simulink model "HumanActionModel"  (R2022b)
settings: Solver=VariableStepAuto  StartTime=0.0  StopTime=5  FixedStep=0.01  RelTol=1e-3
values from neighbouring files (symbols this model uses):
  uD = -0.1    [kavya.mat]
settings Model: Creator=abane  LastModifiedBy=chand

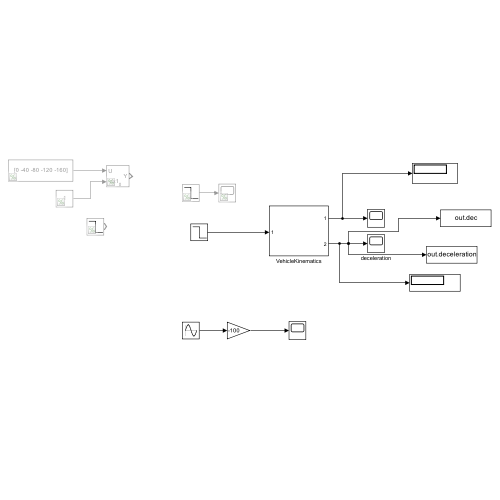
[thumbnail: Simulink's stored preview of the top-level diagram]
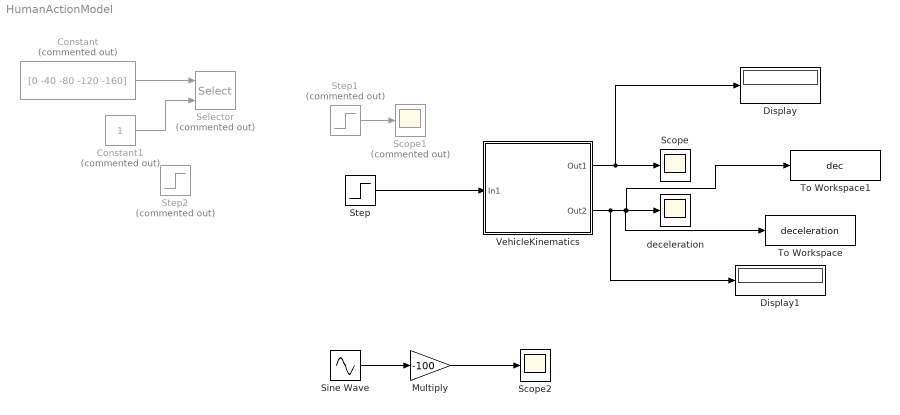
== system HumanActionModel ==
  Constant : Constant  Commented=on  Value=[0 -40 -80 -120 -160]
  Constant1 : Constant  Commented=on
  Display : Display
  Display1 : Display
  Multiply : Gain  Gain=-100
  Scope : Scope
  Scope1 : Scope  Commented=on
  Scope2 : Scope
  Selector : Selector  Commented=on  IndexMode=Zero-based  InputPortWidth=5  IndexOptions=Index vector (port)  Indices=[1 3]  OutputSizes=1
  Sine Wave : Sin  Amplitude=0.5  SampleTime=0
  Step : Step  Time=0.40692  After=-165  SampleTime=0
  Step1 : Step  Commented=on  Time=0.03461  After=-165  SampleTime=0
  Step2 : Step  Commented=on  Time=0.03461  After=-165  SampleTime=0
  To Workspace : ToWorkspace  VariableName=deceleration  SaveFormat=Structure With Time  SampleTime=-1
  To Workspace1 : ToWorkspace  VariableName=dec  SaveFormat=Structure With Time  SampleTime=-1
  VehicleKinematics : Subsystem
  deceleration : Scope
  wires:
  VehicleKinematics/1(Out1) -> Display/1, Scope/1
  VehicleKinematics/2(Out2) -> To Workspace/1, To Workspace1/1, deceleration/1, Display1/1
  Constant/1 -> Selector/1
  Constant1/1 -> Selector/2
  Sine Wave/1 -> Multiply/1
  Multiply/1 -> Scope2/1
  Step/1 -> VehicleKinematics/1(In1)
  Step1/1 -> Scope1/1

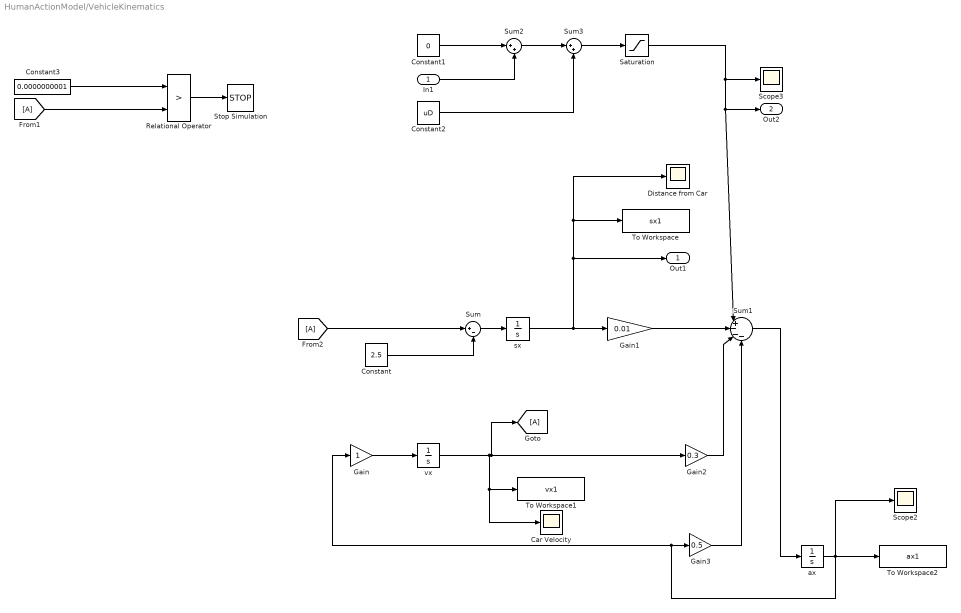
== system HumanActionModel/VehicleKinematics ==
  In1 : Inport
  Car Velocity : Scope
  Constant : Constant  Value=2.5
  Constant1 : Constant  Value=0
  Constant2 : Constant  Value=uD
  Constant3 : Constant  Value=0.0000000001
  Distance from Car : Scope
  From1 : From
  From2 : From
  Gain : Gain
  Gain1 : Gain  Gain=0.01
  Gain2 : Gain  Gain=0.3
  Gain3 : Gain  Gain=0.5
  Goto : Goto
  Relational Operator : RelationalOperator  Operator=>  OutDataTypeStr=boolean  RndMeth=Simplest  InputSameDT=off
  Saturation : Saturate  UpperLimit=0  LowerLimit=-165
  Scope2 : Scope
  Scope3 : Scope
  Stop Simulation : Stop
  Sum : Sum  Inputs=|+-
  Sum1 : Sum  Inputs=|+---
  Sum2 : Sum  Inputs=|++
  Sum3 : Sum  Inputs=|++
  To Workspace : ToWorkspace  VariableName=sx1  SaveFormat=Timeseries  SampleTime=-1
  To Workspace1 : ToWorkspace  VariableName=vx1  SaveFormat=Timeseries  SampleTime=-1
  To Workspace2 : ToWorkspace  VariableName=ax1  SaveFormat=Timeseries  SampleTime=-1
  ax : Integrator
  sx : Integrator  InitialCondition=-43.8
  vx : Integrator  InitialCondition=60
  Out1 : Outport
  Out2 : Outport  Port=2
  wires:
  Constant3/1 -> Relational Operator/1
  Relational Operator/1 -> Stop Simulation/1
  Sum/1 -> sx/1
  Gain/1 -> vx/1
  Constant1/1 -> Sum2/1
  Gain2/1 -> Sum1/3
  In1/1 -> Sum2/2
  ax/1 -> Scope2/1, To Workspace2/1, Gain/1, Gain3/1
  Sum2/1 -> Sum3/1
  sx/1 -> Distance from Car/1, To Workspace/1, Out1/1, Gain1/1
  Sum1/1 -> ax/1
  Gain3/1 -> Sum1/4
  vx/1 -> Car Velocity/1, To Workspace1/1, Goto/1, Gain2/1
  Gain1/1 -> Sum1/2
  Constant2/1 -> Sum3/2
  Constant/1 -> Sum/2
  Sum3/1 -> Saturation/1
  From1/1 -> Relational Operator/2
  From2/1 -> Sum/1
  Saturation/1 -> Sum1/1, Out2/1, Scope3/1
